simulink model "One_Sensor_Simulation"  (R2021a)
settings: Solver=FixedStepAuto  StartTime=0.0  StopTime=200  FixedStep=Ts  RelTol=1e-5
values from neighbouring files (symbols this model uses):
  accel_filter_coef = [    0.0264    0.1405    0.3331    0.3331    0.1405    0.0264]    [quad_params_ekf.m]
  g = ref_acc(3)    [ekf_measurement_jacobian.m]    (also in quad_params_ekf.m = 9.81)
  gyro_filter_den = [ 1.0000    2.2287    2.5245    1.5773    0.5410    0.0796]    [quad_params_ekf.m]
  gyro_filter_num = [ 0.2821    1.2725    2.4208    2.4208    1.2725    0.2821]    [quad_params_ekf.m]
  I = [     0.005831943165131                   0                   0 ... (first row only)    [quad_params_ekf.m]
  Kd_rates = [0.05,0.05,0.1]'    [quad_params_ekf.m]
  Kd_vel = [0.8,0.8,0.3]'    [quad_params_ekf.m]
  Ki_vel = [0.1,0.1,0.1]'    [quad_params_ekf.m]
  km = 1.2e-7    (= 1.2e-07)    [quad_params_ekf.m]
  Kp_att = [6,6,6]'    [quad_params_ekf.m]
  Kp_pos = [7,7,3]'    [quad_params_ekf.m]
  Kp_rates = [10,10,10]'    [quad_params_ekf.m]
  Kp_vel = [3,3,5]'    [quad_params_ekf.m]
  kt = 0.9e-5    (= 9e-06)    [quad_params_ekf.m]
  L = 0.2    [quad_params_ekf.m]
  m = 0.9272    [quad_params_ekf.m]
  q_init = [1;0;0;0]    [quad_params_ekf.m]
  rate_p_max = 3.5    [quad_params_ekf.m]
  thrust_max = thrust_max_per_motor*4    (= 32)    [quad_params_ekf.m]
  thrust_max_per_motor = 8    [quad_params_ekf.m]
  tilt_max = pi/6    (= 0.523598775598)    [quad_params_ekf.m]
  TQ_max_per_motor = km*(w_max.^2)    [quad_params_ekf.m]
  Ts = 0.001    [ekf_process_jacobian.m]    (also in ekf_process_model.m; quad_params_ekf.m)
  Ts_IMU = 0.001    [quad_params_ekf.m]
  Vb_init = [0;0;0]    [quad_params_ekf.m]
  vel_xy_max = 15    [quad_params_ekf.m]
  vel_z_max = 10    [quad_params_ekf.m]
  wb_init = [0;0;0]    [quad_params_ekf.m]
  Xe_init = [0;0;0]    [quad_params_ekf.m]
undefined symbols (not defined in the file or in its folder): IMU, pm_0, sigbuilder_block, Vm_0, xme_0
libraries: simulink_extras x7, aerolibutil x6, sharedutil x5, simulink x4, sharedtransform x4, pid_lib x3, aerolibcommonsys x3, aerolibnavsys x2, mspsensorlib x1, aerolibnav x1, aerolibanim x1
(part 2 of 3)

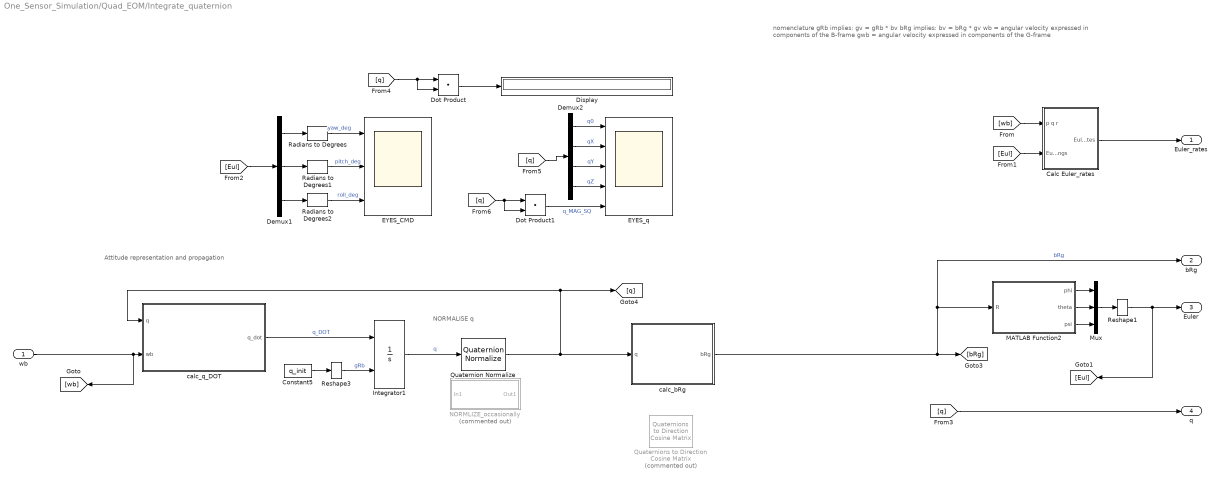
== system One_Sensor_Simulation/Quad_EOM/Integrate_quaternion ==
  note: Attitude representation and propagation
  note: nomenclature
      | gRb implies: gv = gRb * bv
      | bRg implies: bv = bRg * gv
      |
      | wb = angular velocity expressed in components of the B-frame
      | gwb = angular velocity expressed in components of the G-frame
  note: NORMALISE q
  wb : Inport
  Calc Euler_rates : Subsystem
  Constant5 : Constant  Value=q_init  OutDataTypeStr=Inherit: Inherit via back propagation
  Demux1 : Demux  Outputs=3
  Demux2 : Demux
  Display : Display
  Dot Product : DotProduct  InputSameDT=on  OutDataTypeStr=Inherit: Inherit via internal rule
  Dot Product1 : DotProduct  InputSameDT=on  OutDataTypeStr=Inherit: Inherit via internal rule
  EYES_CMD : Scope  NumInputPorts=3
  EYES_q : Scope  NumInputPorts=5
  Integrator1 : Integrator  InitialConditionSource=external
  MATLAB Function2 : MATLAB Function  TreatAsAtomicUnit=on
  Mux : Mux  Inputs=3
  NORMLIZE_occasionally : Subsystem  Commented=on
  Quaternion Normalize : sharedutil/Quaternion Normalize  aMode=aMode
      settings: SourceProductBaseCode=AE,PW,DR,MT,UV,VE
  Quaternions to Direction Cosine Matrix : sharedtransform/Quaternions to  Direction Cosine Matrix  Commented=on  aMode=aMode
      settings: SourceProductBaseCode=AE,PW,DR,MT,UV,VE
  Radians to Degrees : simulink_extras/Transformations/Radians to Degrees
  Radians to Degrees1 : simulink_extras/Transformations/Radians to Degrees
  Radians to Degrees2 : simulink_extras/Transformations/Radians to Degrees
  Reshape1 : Reshape  OutputDimensionality=Column vector (2-D)
  Reshape3 : Reshape  OutputDimensionality=Column vector (2-D)
  calc_bRg : MATLAB Function  TreatAsAtomicUnit=on
  calc_q_DOT : MATLAB Function  TreatAsAtomicUnit=on
  Euler_rates : Outport
  bRg : Outport  Port=2
  Euler : Outport  Port=3
  q : Outport  Port=4
  wires:
  Calc Euler_rates/1(Euler_rates) -> Euler_rates/1
  [Eul] -> Demux1/1
  Demux1/2 -> Radians to Degrees1/1
  Demux1/3 -> Radians to Degrees2/1
  Radians to Degrees2/1 -> EYES_CMD/3  "roll_deg"
  Radians to Degrees1/1 -> EYES_CMD/2  "pitch_deg"
  Radians to Degrees/1 -> EYES_CMD/1  "yaw_deg"
  Demux1/1 -> Radians to Degrees/1
  [Eul] -> Calc Euler_rates/2(Euler_angs)
  [wb] -> Calc Euler_rates/1("p q r ")
  Reshape1/1 -> [Eul], Euler/1
  Mux/1 -> Reshape1/1
  MATLAB Function2/3(psi) -> Mux/3
  MATLAB Function2/2(theta) -> Mux/2
  MATLAB Function2/1(phi) -> Mux/1
  Demux2/3 -> EYES_q/3  "qY"
  [q] -> Demux2/1
  Demux2/2 -> EYES_q/2  "qX"
  Demux2/1 -> EYES_q/1  "q0"
  [q] -> Dot Product1/2, Dot Product1/1
  Demux2/4 -> EYES_q/4  "qZ"
  Dot Product1/1 -> EYES_q/5  "q_MAG_SQ"
  Dot Product/1 -> Display/1
  [q] -> Dot Product/2, Dot Product/1
  Integrator1/1 -> Quaternion Normalize/1  "q"
  Quaternion Normalize/1 -> calc_bRg/1(q), [q], calc_q_DOT/1(q)
  calc_bRg/1(bRg) -> bRg/1, MATLAB Function2/1(R), [bRg]  "bRg"
  calc_q_DOT/1(q_dot) -> Integrator1/1  "q_DOT"
  Constant5/1 -> Reshape3/1
  wb/1 -> calc_q_DOT/2(wb), [wb]
  Reshape3/1 -> Integrator1/2  "gRb"
  [q] -> q/1

== system One_Sensor_Simulation/Quad_EOM/Subsystem ==
  note: I . w^' = Mb - (\omega \times (I.w))
      |
      | w^' = inv(I) * (Mb - (w \times (I.w)))
  pqr : Inport
  I : Inport  Port=2
  Moment : Inport  Port=3
  Product2 : Product  Multiplication=Matrix(*)  InputSameDT=on  SaturateOnIntegerOverflow=on  OutDataTypeStr=Inherit: Same as first input
  Product3 : Product  Inputs=/  Multiplication=Matrix(*)  SaturateOnIntegerOverflow=on  OutDataTypeStr=Inherit: Same as first input
  Product4 : Product  Multiplication=Matrix(*)  SaturateOnIntegerOverflow=on  OutDataTypeStr=Inherit: Same as first input
  Reshape10 : Reshape  OutputDimensionality=Column vector (2-D)
  Reshape8 : Reshape  OutputDimensionality=Column vector (2-D)
  Reshape9 : Reshape  OutputDimensionality=Column vector (2-D)
  Scope : Scope
  Scope1 : Scope
  Scope2 : Scope
  Sum2 : Sum  Inputs=+|-  SaturateOnIntegerOverflow=on
  w_x_(I.w) : Subsystem
      mask Display:
      | text(.5,.5,'Cross\nProduct\n\nC = AxB', ...
      | 	'HorizontalAlignment','Center',...
      | 	'VerticalAlignment','middle')
  pdot qdot rdot : Outport
  wires:
  Product2/1 -> Scope1/1, w_x_(I.w)/2(B)  "I.w"
  Product3/1 -> Product4/1  "inv(I)"
  Reshape8/1 -> Scope/1, w_x_(I.w)/1(A), Product2/2  "w"
  [I] -> Product3/1
  pqr/1 -> Reshape8/1
  Reshape9/1 -> Sum2/1  "Mb"
  Sum2/1 -> Scope2/1, Product4/2  "Mb - (w x (I.w))"
  Reshape10/1 -> Sum2/2  "w x (I.w)"
  w_x_(I.w)/1(C) -> Reshape10/1
  [I] -> Product2/1  "I"
  Product4/1 -> pdot qdot rdot/1  "w_dot"
  Moment/1 -> Reshape9/1
  I/1 -> [I]

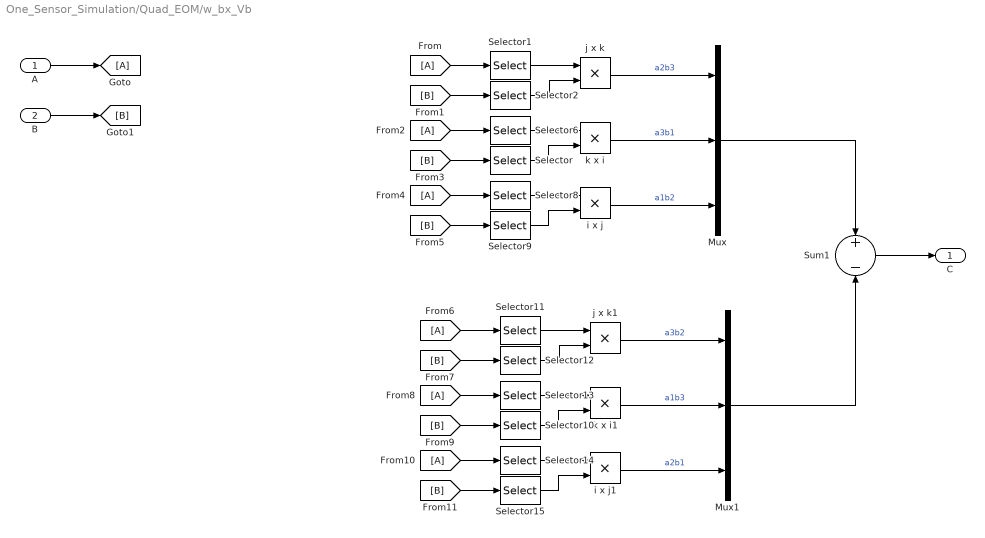
== system One_Sensor_Simulation/Quad_EOM/w_bx_Vb ==
  A : Inport
  B : Inport  Port=2
  Mux : Mux  Inputs=3
  Mux1 : Mux  Inputs=3
  Selector{,8,13,15} (4 alike) : Selector  InputPortWidth=3  IndexOptions=Index vector (dialog)  Indices=1  OutputSizes=1
  Selector{1,9,12,14} (4 alike) : Selector  InputPortWidth=3  IndexOptions=Index vector (dialog)  Indices=2  OutputSizes=1
  Selector{2,6,10..11} (4 alike) : Selector  InputPortWidth=3  IndexOptions=Index vector (dialog)  Indices=3  OutputSizes=1
  Sum1 : Sum  Inputs=+|-  InputSameDT=on  SaturateOnIntegerOverflow=on  OutDataTypeStr=Inherit: Same as first input
  i x j : Product  InputSameDT=on  SaturateOnIntegerOverflow=on  OutDataTypeStr=Inherit: Same as first input
  i x j1 : Product  InputSameDT=on  SaturateOnIntegerOverflow=on  OutDataTypeStr=Inherit: Same as first input
  j x k : Product  InputSameDT=on  SaturateOnIntegerOverflow=on  OutDataTypeStr=Inherit: Same as first input
  j x k1 : Product  InputSameDT=on  SaturateOnIntegerOverflow=on  OutDataTypeStr=Inherit: Same as first input
  k x i : Product  InputSameDT=on  SaturateOnIntegerOverflow=on  OutDataTypeStr=Inherit: Same as first input
  k x i1 : Product  InputSameDT=on  SaturateOnIntegerOverflow=on  OutDataTypeStr=Inherit: Same as first input
  C : Outport
  wires:
  i x j/1 -> Mux/3  "a1b2"
  k x i/1 -> Mux/2  "a3b1"
  j x k/1 -> Mux/1  "a2b3"
  Mux/1 -> Sum1/1
  Sum1/1 -> C/1
  Selector1/1 -> j x k/1
  Selector2/1 -> j x k/2
  B/1 -> [B]
  A/1 -> [A]
  [B] -> Selector2/1
  [A] -> Selector1/1
  [A] -> Selector6/1
  [B] -> Selector/1
  Selector6/1 -> k x i/1
  Selector/1 -> k x i/2
  [A] -> Selector8/1
  [B] -> Selector9/1
  Selector8/1 -> i x j/1
  Selector9/1 -> i x j/2
  i x j1/1 -> Mux1/3  "a2b1"
  k x i1/1 -> Mux1/2  "a1b3"
  j x k1/1 -> Mux1/1  "a3b2"
  Mux1/1 -> Sum1/2
  Selector11/1 -> j x k1/1
  Selector12/1 -> j x k1/2
  [B] -> Selector12/1
  [A] -> Selector11/1
  [A] -> Selector13/1
  [B] -> Selector10/1
  Selector13/1 -> k x i1/1
  Selector10/1 -> k x i1/2
  [A] -> Selector14/1
  [B] -> Selector15/1
  Selector14/1 -> i x j1/1
  Selector15/1 -> i x j1/2

== system One_Sensor_Simulation/Sensors and preprocessing/IMU+altitude ==
  note: Accelerometer and Gyroscope
  note: Magnetometer
  note: Altitude (not simulated)
  States : Inport
  Acc + Gyro : Subsystem  AncestorBlock=aerolibnav/Three-axis Inertial Measurement Unit  mask(Three-axis Inertial Measurement Unit){units=Metric (MKS), imu=[0 0 0], i_Ts=Ts, dtype_a=off, w_a=.7, z_a=.2, a_sf_cc=IMU.accScaleCross, a_bias=IMU.accBias, a_sat=IMU.accLimits, dtype_g=off, w_g=.7, z_g=.2, g_sf_cc=IMU.gyroScaleCross, g_bias=IMU.gyroBias, g_sens=[0, 0, 0], g_sat=IMU.gyroLimits, i_rand=on, i_seeds=IMU.noiseSeeds, i_pow=IMU.noisePower}
      mask prompts: units "aeroblks:aeroblknav:blockThreeaxisInertialMeasurementUnitParamUnits"; imu "aeroblks:aeroblknav:blockThreeaxisInertialMeasurementUnitParamIMUlocation"; i_Ts "aeroblks:aeroblknav:blockThreeaxisInertialMeasurementUnitParamUpdaterate"; dtype_a "aeroblks:aeroblknav:blockThreeaxisInertialMeasurementUnitParamSecondorderdynamicsforaccelerometer"; w_a "aeroblks:aeroblknav:blockThreeaxisInertialMeasurementUnitParamAccelerometernaturalfrequencyradsec"; z_a "aeroblks:aeroblknav:blockThreeaxisInertialMeasurementUnitParamAccelerometerdampingratio"; a_sf_cc "aeroblks:aeroblknav:blockThreeaxisInertialMeasurementUnitParamAccelerometerscalefactorandcrosscoupling"; a_bias "aeroblks:aeroblknav:blockThreeaxisInertialMeasurementUnitParamAccelerometermeasurementbias"; a_sat "aeroblks:aeroblknav:blockThreeaxisInertialMeasurementUnitParamAccelerometerupperandlowerlimits"; dtype_g "aeroblks:aeroblknav:blockThreeaxisInertialMeasurementUnitParamSecondorderdynamicsforgyro"; w_g "aeroblks:aeroblknav:blockThreeaxisInertialMeasurementUnitParamGyronaturalfrequencyradsec"; z_g "aeroblks:aeroblknav:blockThreeaxisInertialMeasurementUnitParamGyrodampingratio"; g_sf_cc "aeroblks:aeroblknav:blockThreeaxisInertialMeasurementUnitParamGyroscalefactorsandcrosscoupling"; g_bias "aeroblks:aeroblknav:blockThreeaxisInertialMeasurementUnitParamGyromeasurementbias"; g_sens "aeroblks:aeroblknav:blockThreeaxisInertialMeasurementUnitParamGsensitivebias"; g_sat "aeroblks:aeroblknav:blockThreeaxisInertialMeasurementUnitParamGyroupperandlowerlimits"; i_rand "aeroblks:aeroblknav:blockThreeaxisInertialMeasurementUnitParamNoiseon"; i_seeds "aeroblks:aeroblknav:blockThreeaxisInertialMeasurementUnitParamNoiseseeds"; i_pow "aeroblks:aeroblknav:blockThreeaxisInertialMeasurementUnitParamNoisepower"
      mask help: aeroblks:aeroblknav:blockThreeaxisInertialMeasurementUnitDesc
      mask init:
      | block = gcb;   
      | ports=aeroicon('aeroblkimu','icon');
      mask Help: eval('asbhelp');
      mask TypeOptions units: aeroblks:aeroblknav:blockThreeaxisInertialMeasurementUnitParamComboMetricMKS | aeroblks:aeroblknav:blockThreeaxisInertialMeasurementUnitParamComboEnglish
      mask Callback dtype_a: aeroicon('aeroblkimu')
      mask Callback dtype_g: aeroicon('aeroblkimu')
      mask Callback i_rand: aeroicon('aeroblkimu')
      mask DialogControl ParameterTabVar0 Prompt: Main
      mask DialogControl units Prompt: Units:
      mask DialogControl imu Prompt: IMU location:
      mask DialogControl i_Ts Prompt: Update rate:
      mask DialogControl ParameterTabVar01 Prompt: Accelerometer
      mask DialogControl dtype_a Prompt: Second-order dynamics for accelerometer
      mask DialogControl w_a Prompt: Accelerometer natural frequency (rad/sec):
      mask DialogControl z_a Prompt: Accelerometer damping ratio:
      mask DialogControl a_sf_cc Prompt: Accelerometer scale factor and cross-coupling:
      mask DialogControl a_bias Prompt: Accelerometer measurement bias:
      mask DialogControl a_sat Prompt: Accelerometer upper and lower limits:
      mask DialogControl ParameterTabVar012 Prompt: Gyroscope
      mask DialogControl dtype_g Prompt: Second-order dynamics for gyro
      mask DialogControl w_g Prompt: Gyro natural frequency (rad/sec):
      mask DialogControl z_g Prompt: Gyro damping ratio:
      mask DialogControl g_sf_cc Prompt: Gyro scale factors and cross-coupling:
      mask DialogControl g_bias Prompt: Gyro measurement bias:
      mask DialogControl g_sens Prompt: G-sensitive bias:
      mask DialogControl g_sat Prompt: Gyro upper and lower limits:
      mask DialogControl ParameterTabVar0123 Prompt: Noise
      mask DialogControl i_rand Prompt: Noise on
      mask DialogControl i_seeds Prompt: Noise seeds:
      mask DialogControl i_pow Prompt: Noise power:
      mask Display:
      | port_label(ports(1).type,ports(1).port,ports(1).txt,'texmode','on');
      | port_label(ports(2).type,ports(2).port,ports(2).txt,'texmode','on');
      | port_label(ports(3).type,ports(3).port,ports(3).txt,'texmode','on');
      | port_label(ports(4).type,ports(4).port,ports(4).txt,'texmode','on');
      | port_label(ports(5).type,ports(5).port,ports(5).txt,'texmode','on');
      | port_label(ports(6).type,ports(6).port,ports(6).txt,'texmode','on');
      | port_label(ports(7).type,ports(7).port,ports(7).txt,'texmode','on');
  Bus Selector : BusSelector  OutputSignals=Ab,wb,wb_dot
  Bus Selector1 : BusSelector  OutputSignals=Ab,bRg
  Bus Selector3 : BusSelector  OutputSignals=phi; theta; psi
  Bus Selector4 : BusSelector  OutputSignals=Xe
  Bus Selector5 : BusSelector  OutputSignals=Ab
  CG location : Constant  Value=[0, 0, 0]
  Compare yaw from mag and actual one : MATLAB Function  TreatAsAtomicUnit=on
  Gravity : Constant  Value=[0 0 -g]
  IMU : mspsensorlib/IMU  Commented=on  DispRefFrame=NED  Temperature=25  MagneticFieldNED=[ 27.5550, -2.4169, -16.0849 ]  MagneticFieldENU=[ -2.4169, 27.5550, 16.0849 ]  SeedDouble=67  SimulateUsing=Interpreted execution  AccelParamsMeasurementRange=Inf  AccelParamsResolution=0  AccelParamsConstantBias=[ 0, 0, 0 ]  AccelParamsAxesMisalignment=[ 0, 0, 0 ]  AccelParamsNoiseDensity=[ 0, 0, 0 ]  AccelParamsBiasInstability=[ 0, 0, 0 ]  AccelParamsRandomWalk=[ 0, 0, 0 ]  AccelParamsTemperatureBias=[ 0, 0, 0 ]  AccelParamsTemperatureScaleFactor=[ 0, 0, 0 ]  GyroParamsMeasurementRange=Inf  GyroParamsResolution=0  GyroParamsConstantBias=[ 0, 0, 0 ]  GyroParamsAxesMisalignment=[ 0, 0, 0 ]  GyroParamsAccelerationBias=[ 0, 0, 0 ]  GyroParamsNoiseDensity=[ 0, 0, 0 ]  GyroParamsBiasInstability=[ 0, 0, 0 ]  GyroParamsRandomWalk=[ 0, 0, 0 ]  GyroParamsTemperatureBias=[ 0, 0, 0 ]  GyroParamsTemperatureScaleFactor=[ 0, 0, 0 ]  MagParamsMeasurementRange=Inf  MagParamsResolution=0  MagParamsConstantBias=[ 0, 0, 0 ]  MagParamsAxesMisalignment=[ 0, 0, 0 ]  MagParamsNoiseDensity=[ 0, 0, 0 ]  MagParamsBiasInstability=[ 0, 0, 0 ]  MagParamsRandomWalk=[ 0, 0, 0 ]  MagParamsTemperatureBias=[ 0, 0, 0 ]  MagParamsTemperatureScaleFactor=[ 0, 0, 0 ]
      settings: SourceProductBaseCode=TF,NV
  Magnetometer : Subsystem
  Mux : Mux  Inputs=2
  Scope : Scope
  Selector : Selector  InputPortWidth=3  IndexOptions=Index vector (dialog)  Indices=[3]  OutputSizes=1
  Selector2 : Selector  InputPortWidth=3  IndexOptions=Index vector (dialog)  Indices=[3]  OutputSizes=1
  Three-axis Inertial Measurement Unit1 : aerolibnav/Three-axis Inertial Measurement Unit  Commented=on  units=Metric (MKS)  imu=[0 0 0]  i_Ts=Ts_IMU  dtype_a=on  w_a=190  z_a=0.707  a_sf_cc=[1 0 0; 0 1 0; 0 0 1]  a_bias=[0 0 0]  a_sat="[-inf  -inf  -inf  inf inf inf]"  dtype_g=on  w_g=190  z_g=0.707  g_sf_cc=[1 0 0; 0 1 0; 0 0 1]  g_bias=[0 0 0]  g_sens=[0 0 0]  g_sat="[-inf  -inf  -inf  inf inf inf]"  i_rand=on  i_seeds=[23093 23094 23095 23096 23097 23098]  i_pow=[0.001 0.001 0.001 0.0001 0.0001 0.0001]
  acc : Outport
  gyro : Outport  Port=2
  alt : Outport  Port=3
  mag : Outport  Port=4
  wires:
  Selector2/1 -> alt/1  "altitude"
  CG location/1 -> Acc + Gyro/4(CG)
  Bus Selector/3 -> Acc + Gyro/3(w_dot)  "<wb_dot>"
  Bus Selector/2 -> Acc + Gyro/2(w)  "<wb>"
  Bus Selector/1 -> Acc + Gyro/1(A_b)  "<Ab>"
  Acc + Gyro/2(w_meas) -> gyro/1  "gyro"
  Gravity/1 -> Acc + Gyro/5(g)  "Gravity_ned"
  Acc + Gyro/1(A_meas) -> acc/1  "acc"
  Selector/1 -> Mux/2  "yaw"
  Compare yaw from mag and actual one/1(yaw) -> Mux/1
  Mux/1 -> Scope/1
  Bus Selector1/2 -> Magnetometer/2(<bRg>)  "<bRg>"
  Magnetometer/1(mag) -> mag/1, Compare yaw from mag and actual one/2(mag_vec)
  States/1 -> [states]
  [states] -> Bus Selector/1
  [states] -> Bus Selector1/1
  [states] -> Bus Selector3/1
  Bus Selector3/1 -> Selector/1  "<phi; theta; psi>"
  [states] -> Bus Selector4/1
  Bus Selector4/1 -> Selector2/1  "<Xe>"
  Bus Selector1/1 -> Magnetometer/1(acc)  "<Ab>"
  [states] -> Bus Selector5/1
  Bus Selector5/1 -> Compare yaw from mag and actual one/1(acc_vec)  "<Ab>"

== system One_Sensor_Simulation/Sensors and preprocessing/Preprocessing and Filtering ==
  acc_raw : Inport
  gyro_raw : Inport  Port=2
  alt_raw : Inport  Port=3
  mag_raw : Inport  Port=4
  Cast To Double{,1..2,4} (4 alike) : DataTypeConversion  OutDataTypeStr=double
  Constant : Constant  Value=[0 0 g]
  FIR_IMUaccel : DiscreteFir  Coefficients=accel_filter_coef
  IIR_IMUgyro : DiscreteFilter  Numerator=gyro_filter_num  Denominator=gyro_filter_den
  Sum : Sum  Inputs=-+|
  Sum1 : Sum  Inputs=-+|
  Sum2 : Sum  Inputs=-+|
  Sum3 : Sum  Inputs=|+-
  bias : Constant  Value=IMU.accBiasEst
  filtering : Subsystem
  gyro bias : Constant  Value=IMU.gyroBiasEst
  inverseI_acc_gain : Gain  Gain=IMU.inverseAccGain  ParamDataTypeStr=single  OutDataTypeStr=single
  inverseI_gyro_gain : Gain  Gain=IMU.inverseGyroGain  ParamDataTypeStr=single  OutDataTypeStr=single
  inverseI_mag_gain : Gain  Gain=IMU.inverseMagGain  ParamDataTypeStr=single  OutDataTypeStr=single
  mag bias : Constant  Value=IMU.magBiasEst
  acc_zero : Outport
  acc : Outport  Port=2
  gyro : Outport  Port=3
  alt : Outport  Port=4
  mag : Outport  Port=5
  wires:
  gyro bias/1 -> Sum2/1
  Cast To Double/1 -> acc/1, Sum/2  "acc"
  bias/1 -> Sum1/1
  mag bias/1 -> Sum3/2
  FIR_IMUaccel/1 -> Cast To Double/1  "acc"
  inverseI_gyro_gain/1 -> filtering/1(gyro_raw)  "gyro"
  mag_raw/1 -> Sum3/1
  Sum3/1 -> inverseI_mag_gain/1  "gyro"
  Sum1/1 -> inverseI_acc_gain/1  "acc"
  Sum/1 -> acc_zero/1  "acc_zero"
  Sum2/1 -> inverseI_gyro_gain/1  "gyro"
  Cast To Double1/1 -> gyro/1  "gyro"
  inverseI_mag_gain/1 -> IIR_IMUgyro/1  "mag"
  IIR_IMUgyro/1 -> Cast To Double4/1
  filtering/1(gyro) -> Cast To Double1/1  "gyro"
  inverseI_acc_gain/1 -> FIR_IMUaccel/1  "acc"
  Cast To Double4/1 -> mag/1  "mag"
  Constant/1 -> Sum/1
  acc_raw/1 -> Sum1/2
  gyro_raw/1 -> Sum2/2
  Cast To Double2/1 -> alt/1  "alt"
  alt_raw/1 -> Cast To Double2/1

== system One_Sensor_Simulation/Trajectory command/Altitude ==
  "Altitude " : Subsystem  Tag=STV Subsys  LoadFcn=sigbuilder_block('load');  StartFcn=sigbuilder_block('start');  StopFcn=sigbuilder_block('stop');  ClipboardFcn=sigbuilder_block('clipboard');  VariantControl=Choice_1  mask(Sigbuilder block){tuvar=[0:10]}
      mask help: Simulink:masks:SigbuilderBlock_MD
      mask init:
      | if ~strcmp(get_param(bdroot(gcbh),'SimulationStatus'),'stopped') tuvar = sigbuilder_block('maskInit'); end
      settings: CopyFcn=sigbuilder_block('copy');  DeleteFcn=sigbuilder_block('delete');  ModelCloseFcn=sigbuilder_block('modelClose');  PreSaveFcn=sigbuilder_block('preSave');  PauseFcn=sigbuilder_block('pause');  ContinueFcn=sigbuilder_block('continue');  NameChangeFcn=sigbuilder_block('namechange');  OpenFcn=sigbuilder_block('open',[200.1 155.1 551.4 400.5 ]);  CloseFcn=sigbuilder_block('close');
      mask Display: plot(0, 0, 100, 100,[2, 2, 32, 32, 2], [68, 8, 8, 68, 68],[32, 2], [38, 38], [32, 19, 2],[53, 60, 44], [32, 17, 17, 2],[16, 16, 31, 31]);txt = getActiveGroup(gcbh);text(2, 100, txt,'verticalAlignment', 'top');
  Bus Creator : BusCreator  Inputs=4
  Z : Outport
  Y : Outport  Port=2
  X : Outport  Port=3
  Yaw : Outport  Port=4
  CMD_VEC : Outport  Port=5
  wires:
  "Altitude "/4(Yaw) -> Bus Creator/1, Yaw/1  "yaw_cmd"
  "Altitude "/2(Y) -> Bus Creator/3, Y/1  "y_cmd"
  "Altitude "/1(Z) -> Bus Creator/4, Z/1  "z_cmd"
  "Altitude "/3(X) -> Bus Creator/2, X/1  "x_cmd"
  Bus Creator/1 -> CMD_VEC/1

== system One_Sensor_Simulation/Trajectory command/Ground ==
  Bus Creator : BusCreator  Inputs=4
  Zero{,1..3} (4 alike) : Constant  Value=0  OutDataTypeStr=Inherit: Inherit via back propagation
  Z : Outport
  Y : Outport  Port=2
  X : Outport  Port=3
  Yaw : Outport  Port=4
  CMD_VEC : Outport  Port=5
  wires:
  Zero3/1 -> Bus Creator/1, Yaw/1  "yaw_cmd"
  Zero2/1 -> Bus Creator/3, Y/1  "y_cmd"
  Zero/1 -> Bus Creator/4, Z/1  "z_cmd"
  Zero1/1 -> Bus Creator/2, X/1  "x_cmd"
  Bus Creator/1 -> CMD_VEC/1

== system One_Sensor_Simulation/Trajectory command/Position Trajectory ==
  Bus Creator : BusCreator  Inputs=4
  Degrees to Radians : simulink_extras/Transformations/Degrees to Radians
  multisteps : Subsystem  Tag=STV Subsys  LoadFcn=sigbuilder_block('load');  StartFcn=sigbuilder_block('start');  StopFcn=sigbuilder_block('stop');  ClipboardFcn=sigbuilder_block('clipboard');  VariantControl=Choice_5  mask(Sigbuilder block){tuvar=[0:10]}
      mask help: Simulink:masks:SigbuilderBlock_MD
      mask init:
      | if ~strcmp(get_param(bdroot(gcbh),'SimulationStatus'),'stopped') tuvar = sigbuilder_block('maskInit'); end
      settings: CopyFcn=sigbuilder_block('copy');  DeleteFcn=sigbuilder_block('delete');  ModelCloseFcn=sigbuilder_block('modelClose');  PreSaveFcn=sigbuilder_block('preSave');  PauseFcn=sigbuilder_block('pause');  ContinueFcn=sigbuilder_block('continue');  NameChangeFcn=sigbuilder_block('namechange');  OpenFcn=sigbuilder_block('open',[4.8 36 1142.4 525.6 ]);  CloseFcn=sigbuilder_block('close');
      mask Display: plot(0, 0, 100, 100,[2, 2, 32, 32, 2], [68, 8, 8, 68, 68],[32, 2], [38, 38], [32, 19, 2],[53, 60, 44], [32, 17, 17, 2],[16, 16, 31, 31]);txt = getActiveGroup(gcbh);text(2, 100, txt,'verticalAlignment', 'top');
  Z : Outport
  Y : Outport  Port=2
  X : Outport  Port=3
  Yaw : Outport  Port=4
  CMD_VEC : Outport  Port=5
  wires:
  Degrees to Radians/1 -> Bus Creator/1, Yaw/1  "yaw_cmd"
  multisteps/2(Y) -> Bus Creator/3, Y/1  "y_cmd"
  multisteps/1(Z) -> Bus Creator/4, Z/1  "z_cmd"
  multisteps/3(X) -> Bus Creator/2, X/1  "x_cmd"
  Bus Creator/1 -> CMD_VEC/1
  multisteps/4(Yaw) -> Degrees to Radians/1  "yaw_cmd"

== system One_Sensor_Simulation/Trajectory command/Test to visualize thrust dir ==
  Bus Creator : BusCreator  Inputs=4
  multisteps : Subsystem  Tag=STV Subsys  LoadFcn=sigbuilder_block('load');  StartFcn=sigbuilder_block('start');  StopFcn=sigbuilder_block('stop');  ClipboardFcn=sigbuilder_block('clipboard');  VariantControl=Choice_5  mask(Sigbuilder block){tuvar=[0:10]}
      mask help: Simulink:masks:SigbuilderBlock_MD
      mask init:
      | if ~strcmp(get_param(bdroot(gcbh),'SimulationStatus'),'stopped') tuvar = sigbuilder_block('maskInit'); end
      settings: CopyFcn=sigbuilder_block('copy');  DeleteFcn=sigbuilder_block('delete');  ModelCloseFcn=sigbuilder_block('modelClose');  PreSaveFcn=sigbuilder_block('preSave');  PauseFcn=sigbuilder_block('pause');  ContinueFcn=sigbuilder_block('continue');  NameChangeFcn=sigbuilder_block('namechange');  OpenFcn=sigbuilder_block('open',[0 36 1152 560.4 ]);  CloseFcn=sigbuilder_block('close');
      mask Display: plot(0, 0, 100, 100,[2, 2, 32, 32, 2], [68, 8, 8, 68, 68],[32, 2], [38, 38], [32, 19, 2],[53, 60, 44], [32, 17, 17, 2],[16, 16, 31, 31]);txt = getActiveGroup(gcbh);text(2, 100, txt,'verticalAlignment', 'top');
  Z : Outport
  Y : Outport  Port=2
  X : Outport  Port=3
  Yaw : Outport  Port=4
  CMD_VEC : Outport  Port=5
  wires:
  multisteps/2(Y) -> Bus Creator/3, Y/1  "y_cmd"
  multisteps/1(Z) -> Bus Creator/4, Z/1  "z_cmd"
  multisteps/3(X) -> Bus Creator/2, X/1  "x_cmd"
  Bus Creator/1 -> CMD_VEC/1
  multisteps/4(Yaw) -> Bus Creator/1, Yaw/1  "yaw_cmd"

== system One_Sensor_Simulation/Trajectory command/X Sine ==
  Bus Creator : BusCreator  Inputs=4
  sine wave on X : Subsystem  Tag=STV Subsys  LoadFcn=sigbuilder_block('load');  StartFcn=sigbuilder_block('start');  StopFcn=sigbuilder_block('stop');  ClipboardFcn=sigbuilder_block('clipboard');  VariantControl=Choice_3  mask(Sigbuilder block){tuvar=[0:10]}
      mask help: Simulink:masks:SigbuilderBlock_MD
      mask init:
      | if ~strcmp(get_param(bdroot(gcbh),'SimulationStatus'),'stopped') tuvar = sigbuilder_block('maskInit'); end
      settings: CopyFcn=sigbuilder_block('copy');  DeleteFcn=sigbuilder_block('delete');  ModelCloseFcn=sigbuilder_block('modelClose');  PreSaveFcn=sigbuilder_block('preSave');  PauseFcn=sigbuilder_block('pause');  ContinueFcn=sigbuilder_block('continue');  NameChangeFcn=sigbuilder_block('namechange');  OpenFcn=sigbuilder_block('open',[452.4 149.7 551.4 400.5 ]);  CloseFcn=sigbuilder_block('close');
      mask Display: plot(0, 0, 100, 100,[2, 2, 32, 32, 2], [68, 8, 8, 68, 68],[32, 2], [38, 38], [32, 19, 2],[53, 60, 44], [32, 17, 17, 2],[16, 16, 31, 31]);txt = getActiveGroup(gcbh);text(2, 100, txt,'verticalAlignment', 'top');
  Z : Outport
  Y : Outport  Port=2
  X : Outport  Port=3
  Yaw : Outport  Port=4
  CMD_VEC : Outport  Port=5
  wires:
  sine wave on X/4(Yaw) -> Bus Creator/1, Yaw/1  "yaw_cmd"
  sine wave on X/2(Y) -> Bus Creator/3, Y/1  "y_cmd"
  sine wave on X/1(Z) -> Bus Creator/4, Z/1  "z_cmd"
  sine wave on X/3(X) -> Bus Creator/2, X/1  "x_cmd"
  Bus Creator/1 -> CMD_VEC/1

== system One_Sensor_Simulation/Trajectory command/X ramp ==
  " ramp on X" : Subsystem  Tag=STV Subsys  LoadFcn=sigbuilder_block('load');  StartFcn=sigbuilder_block('start');  StopFcn=sigbuilder_block('stop');  ClipboardFcn=sigbuilder_block('clipboard');  VariantControl=Choice_3  mask(Sigbuilder block){tuvar=[0:10]}
      mask help: Simulink:masks:SigbuilderBlock_MD
      mask init:
      | if ~strcmp(get_param(bdroot(gcbh),'SimulationStatus'),'stopped') tuvar = sigbuilder_block('maskInit'); end
      settings: CopyFcn=sigbuilder_block('copy');  DeleteFcn=sigbuilder_block('delete');  ModelCloseFcn=sigbuilder_block('modelClose');  PreSaveFcn=sigbuilder_block('preSave');  PauseFcn=sigbuilder_block('pause');  ContinueFcn=sigbuilder_block('continue');  NameChangeFcn=sigbuilder_block('namechange');  OpenFcn=sigbuilder_block('open',[76.2 101.7 551.4 400.5 ]);  CloseFcn=sigbuilder_block('close');
      mask Display: plot(0, 0, 100, 100,[2, 2, 32, 32, 2], [68, 8, 8, 68, 68],[32, 2], [38, 38], [32, 19, 2],[53, 60, 44], [32, 17, 17, 2],[16, 16, 31, 31]);txt = getActiveGroup(gcbh);text(2, 100, txt,'verticalAlignment', 'top');
  Bus Creator : BusCreator  Inputs=4
  Z : Outport
  Y : Outport  Port=2
  X : Outport  Port=3
  Yaw : Outport  Port=4
  CMD_VEC : Outport  Port=5
  wires:
  " ramp on X"/4(Yaw) -> Bus Creator/1, Yaw/1  "yaw_cmd"
  " ramp on X"/2(Y) -> Bus Creator/3, Y/1  "y_cmd"
  " ramp on X"/1(Z) -> Bus Creator/4, Z/1  "z_cmd"
  " ramp on X"/3(X) -> Bus Creator/2, X/1  "x_cmd"
  Bus Creator/1 -> CMD_VEC/1

== system One_Sensor_Simulation/Trajectory command/X square ==
  Bus Creator : BusCreator  Inputs=4
  sine wave on X : Subsystem  Tag=STV Subsys  LoadFcn=sigbuilder_block('load');  StartFcn=sigbuilder_block('start');  StopFcn=sigbuilder_block('stop');  ClipboardFcn=sigbuilder_block('clipboard');  VariantControl=Choice_3  mask(Sigbuilder block){tuvar=[0:10]}
      mask help: Simulink:masks:SigbuilderBlock_MD
      mask init:
      | if ~strcmp(get_param(bdroot(gcbh),'SimulationStatus'),'stopped') tuvar = sigbuilder_block('maskInit'); end
      settings: CopyFcn=sigbuilder_block('copy');  DeleteFcn=sigbuilder_block('delete');  ModelCloseFcn=sigbuilder_block('modelClose');  PreSaveFcn=sigbuilder_block('preSave');  PauseFcn=sigbuilder_block('pause');  ContinueFcn=sigbuilder_block('continue');  NameChangeFcn=sigbuilder_block('namechange');  OpenFcn=sigbuilder_block('open',[452.4 149.7 551.4 400.5 ]);  CloseFcn=sigbuilder_block('close');
      mask Display: plot(0, 0, 100, 100,[2, 2, 32, 32, 2], [68, 8, 8, 68, 68],[32, 2], [38, 38], [32, 19, 2],[53, 60, 44], [32, 17, 17, 2],[16, 16, 31, 31]);txt = getActiveGroup(gcbh);text(2, 100, txt,'verticalAlignment', 'top');
  Z : Outport
  Y : Outport  Port=2
  X : Outport  Port=3
  Yaw : Outport  Port=4
  CMD_VEC : Outport  Port=5
  wires:
  sine wave on X/4(Yaw) -> Bus Creator/1, Yaw/1  "yaw_cmd"
  sine wave on X/2(Y) -> Bus Creator/3, Y/1  "y_cmd"
  sine wave on X/1(Z) -> Bus Creator/4, Z/1  "z_cmd"
  sine wave on X/3(X) -> Bus Creator/2, X/1  "x_cmd"
  Bus Creator/1 -> CMD_VEC/1

== system One_Sensor_Simulation/Trajectory command/Y Sine ==
  Bus Creator : BusCreator  Inputs=4
  sine wave on Y : Subsystem  Tag=STV Subsys  LoadFcn=sigbuilder_block('load');  StartFcn=sigbuilder_block('start');  StopFcn=sigbuilder_block('stop');  ClipboardFcn=sigbuilder_block('clipboard');  VariantControl=Choice_3  mask(Sigbuilder block){tuvar=[0:10]}
      mask help: Simulink:masks:SigbuilderBlock_MD
      mask init:
      | if ~strcmp(get_param(bdroot(gcbh),'SimulationStatus'),'stopped') tuvar = sigbuilder_block('maskInit'); end
      settings: CopyFcn=sigbuilder_block('copy');  DeleteFcn=sigbuilder_block('delete');  ModelCloseFcn=sigbuilder_block('modelClose');  PreSaveFcn=sigbuilder_block('preSave');  PauseFcn=sigbuilder_block('pause');  ContinueFcn=sigbuilder_block('continue');  NameChangeFcn=sigbuilder_block('namechange');  OpenFcn=sigbuilder_block('open',[4.8 36 1142.4 525.6 ]);  CloseFcn=sigbuilder_block('close');
      mask Display: plot(0, 0, 100, 100,[2, 2, 32, 32, 2], [68, 8, 8, 68, 68],[32, 2], [38, 38], [32, 19, 2],[53, 60, 44], [32, 17, 17, 2],[16, 16, 31, 31]);txt = getActiveGroup(gcbh);text(2, 100, txt,'verticalAlignment', 'top');
  Z : Outport
  Y : Outport  Port=2
  X : Outport  Port=3
  Yaw : Outport  Port=4
  CMD_VEC : Outport  Port=5
  wires:
  sine wave on Y/4(Yaw) -> Bus Creator/1, Yaw/1  "yaw_cmd"
  sine wave on Y/2(Y) -> Bus Creator/3, Y/1  "y_cmd"
  sine wave on Y/1(Z) -> Bus Creator/4, Z/1  "z_cmd"
  sine wave on Y/3(X) -> Bus Creator/2, X/1  "x_cmd"
  Bus Creator/1 -> CMD_VEC/1

== system One_Sensor_Simulation/Trajectory command/Y ramp ==
  Bus Creator : BusCreator  Inputs=4
  square on Y : Subsystem  Tag=STV Subsys  LoadFcn=sigbuilder_block('load');  StartFcn=sigbuilder_block('start');  StopFcn=sigbuilder_block('stop');  ClipboardFcn=sigbuilder_block('clipboard');  VariantControl=Choice_3  mask(Sigbuilder block){tuvar=[0:10]}
      mask help: Simulink:masks:SigbuilderBlock_MD
      mask init:
      | if ~strcmp(get_param(bdroot(gcbh),'SimulationStatus'),'stopped') tuvar = sigbuilder_block('maskInit'); end
      settings: CopyFcn=sigbuilder_block('copy');  DeleteFcn=sigbuilder_block('delete');  ModelCloseFcn=sigbuilder_block('modelClose');  PreSaveFcn=sigbuilder_block('preSave');  PauseFcn=sigbuilder_block('pause');  ContinueFcn=sigbuilder_block('continue');  NameChangeFcn=sigbuilder_block('namechange');  OpenFcn=sigbuilder_block('open',[4.8 36 1142.4 525.6 ]);  CloseFcn=sigbuilder_block('close');
      mask Display: plot(0, 0, 100, 100,[2, 2, 32, 32, 2], [68, 8, 8, 68, 68],[32, 2], [38, 38], [32, 19, 2],[53, 60, 44], [32, 17, 17, 2],[16, 16, 31, 31]);txt = getActiveGroup(gcbh);text(2, 100, txt,'verticalAlignment', 'top');
  Z : Outport
  Y : Outport  Port=2
  X : Outport  Port=3
  Yaw : Outport  Port=4
  CMD_VEC : Outport  Port=5
  wires:
  square on Y/4(Yaw) -> Bus Creator/1, Yaw/1  "yaw_cmd"
  square on Y/2(Y) -> Bus Creator/3, Y/1  "y_cmd"
  square on Y/1(Z) -> Bus Creator/4, Z/1  "z_cmd"
  square on Y/3(X) -> Bus Creator/2, X/1  "x_cmd"
  Bus Creator/1 -> CMD_VEC/1

== system One_Sensor_Simulation/Trajectory command/Yaw Sine ==
  Bus Creator : BusCreator  Inputs=4
  yaw : Subsystem  Tag=STV Subsys  LoadFcn=sigbuilder_block('load');  StartFcn=sigbuilder_block('start');  StopFcn=sigbuilder_block('stop');  ClipboardFcn=sigbuilder_block('clipboard');  VariantControl=Choice_4  mask(Sigbuilder block){tuvar=[0:10]}
      mask help: Simulink:masks:SigbuilderBlock_MD
      mask init:
      | if ~strcmp(get_param(bdroot(gcbh),'SimulationStatus'),'stopped') tuvar = sigbuilder_block('maskInit'); end
      settings: CopyFcn=sigbuilder_block('copy');  DeleteFcn=sigbuilder_block('delete');  ModelCloseFcn=sigbuilder_block('modelClose');  PreSaveFcn=sigbuilder_block('preSave');  PauseFcn=sigbuilder_block('pause');  ContinueFcn=sigbuilder_block('continue');  NameChangeFcn=sigbuilder_block('namechange');  OpenFcn=sigbuilder_block('open',[452.4 149.7 551.4 400.5 ]);  CloseFcn=sigbuilder_block('close');
      mask Display: plot(0, 0, 100, 100,[2, 2, 32, 32, 2], [68, 8, 8, 68, 68],[32, 2], [38, 38], [32, 19, 2],[53, 60, 44], [32, 17, 17, 2],[16, 16, 31, 31]);txt = getActiveGroup(gcbh);text(2, 100, txt,'verticalAlignment', 'top');
  Z : Outport
  Y : Outport  Port=2
  X : Outport  Port=3
  Yaw : Outport  Port=4
  CMD_VEC : Outport  Port=5
  wires:
  yaw/4(Yaw) -> Bus Creator/1, Yaw/1  "yaw_cmd"
  yaw/2(Y) -> Bus Creator/3, Y/1  "y_cmd"
  yaw/1(Z) -> Bus Creator/4, Z/1  "z_cmd"
  yaw/3(X) -> Bus Creator/2, X/1  "x_cmd"
  Bus Creator/1 -> CMD_VEC/1

== system One_Sensor_Simulation/Trajectory command/Yaw steps ==
  Bus Creator : BusCreator  Inputs=4
  yaw steps : Subsystem  Tag=STV Subsys  LoadFcn=sigbuilder_block('load');  StartFcn=sigbuilder_block('start');  StopFcn=sigbuilder_block('stop');  ClipboardFcn=sigbuilder_block('clipboard');  VariantControl=Choice_4  mask(Sigbuilder block){tuvar=[0:10]}
      mask help: Simulink:masks:SigbuilderBlock_MD
      mask init:
      | if ~strcmp(get_param(bdroot(gcbh),'SimulationStatus'),'stopped') tuvar = sigbuilder_block('maskInit'); end
      settings: CopyFcn=sigbuilder_block('copy');  DeleteFcn=sigbuilder_block('delete');  ModelCloseFcn=sigbuilder_block('modelClose');  PreSaveFcn=sigbuilder_block('preSave');  PauseFcn=sigbuilder_block('pause');  ContinueFcn=sigbuilder_block('continue');  NameChangeFcn=sigbuilder_block('namechange');  OpenFcn=sigbuilder_block('open',[452.4 149.7 551.4 400.5 ]);  CloseFcn=sigbuilder_block('close');
      mask Display: plot(0, 0, 100, 100,[2, 2, 32, 32, 2], [68, 8, 8, 68, 68],[32, 2], [38, 38], [32, 19, 2],[53, 60, 44], [32, 17, 17, 2],[16, 16, 31, 31]);txt = getActiveGroup(gcbh);text(2, 100, txt,'verticalAlignment', 'top');
  Z : Outport
  Y : Outport  Port=2
  X : Outport  Port=3
  Yaw : Outport  Port=4
  CMD_VEC : Outport  Port=5
  wires:
  yaw steps/4(Yaw) -> Bus Creator/1, Yaw/1  "yaw_cmd"
  yaw steps/2(Y) -> Bus Creator/3, Y/1  "y_cmd"
  yaw steps/1(Z) -> Bus Creator/4, Z/1  "z_cmd"
  yaw steps/3(X) -> Bus Creator/2, X/1  "x_cmd"
  Bus Creator/1 -> CMD_VEC/1

== system One_Sensor_Simulation/Control allocation and motor control/Ideal Actuators with allocation/Control allocation ==
  note: $C^{-1} = \left(\begin{array}{cccc} \frac{1}{4\,\mathrm{kt}} & 0 & \frac{1}{2\,L\,\mathrm{kt}} & -\frac{1}{4\,\mathrm{km}}\\ \frac{1}{4\,\mathrm{kt}} & -\frac{1}{2\,L\,\mathrm{kt}} & 0 & \frac{1}{4\,\mathrm{km}}\\ \frac{1}{4\,\mathrm{kt}} & 0 & -\frac{1}{2\,L\,\mathrm{kt}} & -\frac{1}{4\,\mathrm{km}}\\ \frac{1}{4\,\mathrm{kt}} & \frac{1}{2\,L\,\mathrm{kt}} & 0 & \frac{1}{4\,\mathrm{km}} \end{array}\right)$
  note: THRUST = k_t . \omega^2
      |
      | TORQUE = k_m . \omega^2
  THRUST_CMD : Inport
  TQ_Roll_CMD : Inport  Port=2
  TQ_Pitch_CMD : Inport  Port=3
  TQ_Yaw_CMD : Inport  Port=4
  CMD F_and_M and wRPS : Scope  NumInputPorts=8
  Constant : Constant  Value=kt
  Constant1 : Constant  Value=km
  Constant2 : Constant  Value=L
  Demux1 : Demux
  Demux2 : Demux
  Demux3 : Demux
  FM_to_w2 : MATLAB Function  TreatAsAtomicUnit=on
  Mux : Mux
  Scope : Scope
  Sqrt : Sqrt  SaturateOnIntegerOverflow=on
  Subsystem : Subsystem
  W2_checker : Subsystem
  w_command : Outport  VectorParamsAs1DForOutWhenUnconnected=off
  wires:
  Constant1/1 -> FM_to_w2/3(km)
  Constant/1 -> FM_to_w2/2(kt)
  Constant2/1 -> FM_to_w2/1(L)
  FM_to_w2/1(w2_cmd) -> Scope/1, W2_checker/1(w2_CMD)
  Sqrt/1 -> w_command/1, [w_CMD]  "w"
  W2_checker/1(w2) -> Sqrt/1
  Demux1/1 -> FM_to_w2/4(Thrust)
  Demux1/2 -> FM_to_w2/5(M_x)
  Demux1/3 -> FM_to_w2/6(M_y)
  Demux1/4 -> FM_to_w2/7(M_z)
  THRUST_CMD/1 -> Mux/1
  TQ_Roll_CMD/1 -> Mux/2
  TQ_Pitch_CMD/1 -> Mux/3
  TQ_Yaw_CMD/1 -> Mux/4
  Mux/1 -> [FM_CMD]
  [FM_CMD] -> Demux1/1
  Demux2/1 -> CMD F_and_M and wRPS/1  "Thrust"
  Demux2/2 -> CMD F_and_M and wRPS/2  "TQ_Roll_X"
  Demux2/3 -> CMD F_and_M and wRPS/3  "TQ_Pitch_Y"
  Demux2/4 -> CMD F_and_M and wRPS/4  "TQ_Yaw_Z"
  Demux3/2 -> CMD F_and_M and wRPS/6  "w2_RPS"
  Demux3/1 -> CMD F_and_M and wRPS/5  "w1_RPS"
  Demux3/4 -> CMD F_and_M and wRPS/8  "w4_RPS"
  Demux3/3 -> CMD F_and_M and wRPS/7  "w3_RPS"
  [FM_CMD] -> Demux2/1
  Subsystem/1(RPS) -> Demux3/1
  [w_CMD] -> Subsystem/1(w_per_sec)

== system One_Sensor_Simulation/Control allocation and motor control/Ideal Actuators with allocation/Perfect actuators ==
  w_cmd : Inport
  Allocation matrix (motor speed to twist) : MATLAB Function  TreatAsAtomicUnit=on
  Constant3 : Constant  Value=kt
  Constant4 : Constant  Value=km
  Constant5 : Constant  Value=L
  Demux : Demux
  Math Function1 : Math  Operator=square  SignedPower=on  SaturateOnIntegerOverflow=on
  Motor Control : Subsystem
      mask Display: image('$imagefile'); % Use "Edit Image" on toolstrip to change.
  Mux1 : Mux
  Reshape1 : Reshape  OutputDimensionality=Column vector (2-D)
  Thrust : Outport  VectorParamsAs1DForOutWhenUnconnected=off
  Mx : Outport  Port=2  VectorParamsAs1DForOutWhenUnconnected=off
  My : Outport  Port=3  VectorParamsAs1DForOutWhenUnconnected=off
  Mz : Outport  Port=4  VectorParamsAs1DForOutWhenUnconnected=off
  T_actual : Outport  Port=5  VectorParamsAs1DForOutWhenUnconnected=off
  w_mot_actual : Outport  Port=6  VectorParamsAs1DForOutWhenUnconnected=off
  wires:
  Demux/2 -> Mx/1
  Demux/1 -> Thrust/1
  Demux/3 -> My/1
  Demux/4 -> Mz/1
  [FM] -> Demux/1
  Constant3/1 -> Allocation matrix (motor speed to twist)/2(kt)
  Mux1/1 -> [FM]
  Allocation matrix (motor speed to twist)/4(M_z) -> Mux1/4
  Allocation matrix (motor speed to twist)/1(Thrust) -> Mux1/1
  Allocation matrix (motor speed to twist)/2(M_x) -> Mux1/2
  Allocation matrix (motor speed to twist)/3(M_y) -> Mux1/3
  Constant4/1 -> Allocation matrix (motor speed to twist)/3(km)
  [FM] -> T_actual/1
  Constant5/1 -> Allocation matrix (motor speed to twist)/1(L)
  Math Function1/1 -> Allocation matrix (motor speed to twist)/4(w2_col)
  Reshape1/1 -> Math Function1/1
  Motor Control/1(w) -> w_mot_actual/1, Reshape1/1  "w_actual"
  w_cmd/1 -> Motor Control/1(w_CMD)

== system One_Sensor_Simulation/Quad with sensors/Integrate_quaternion/Calc Euler_rates ==
  "p q r " : Inport
  Euler_angs : Inport  Port=2
  Demux1 : Demux  Outputs=3
  Demux2 : Demux  Outputs=3
  Demux3 : Demux  Outputs=3
  Mux1 : Mux  Inputs=3
  Reshape1 : Reshape  OutputDimensionality=Column vector (2-D)
  Reshape2 : Reshape  OutputDimensionality=Column vector (2-D)
  Terminator : Terminator
  euler_rates : MATLAB Function  TreatAsAtomicUnit=on
  Euler_rates : Outport
  wires:
  Demux2/2 -> Mux1/2  "thetadot_Y2_pitch"
  Demux1/1 -> euler_rates/1(phi_t)  "phi"
  Demux3/2 -> euler_rates/4(q)
  Demux2/1 -> Mux1/1  "phidot_Z1_yaw"
  "p q r "/1 -> Reshape1/1
  Euler_angs/1 -> Demux1/1
  Demux3/1 -> euler_rates/3(p)
  Reshape2/1 -> Euler_rates/1
  Reshape1/1 -> Demux3/1  "wb"
  Demux3/3 -> euler_rates/5(r)
  Demux1/3 -> Terminator/1  "psi"
  euler_rates/1(euler_rates) -> Demux2/1  "euler_rates"
  Demux1/2 -> euler_rates/2(theta_t)  "theta"
  Mux1/1 -> Reshape2/1
  Demux2/3 -> Mux1/3  "psidot_X3_roll"

== system One_Sensor_Simulation/Quad with sensors/Integrate_quaternion/NORMLIZE_occasionally ==
  note: One strategy for NORMALIZING the quaternion
  note: eg: every 10 seconds normalize
  In1 : Inport
  Adjust_to_UNITY : Subsystem
  Out1 : Outport
  wires:
  In1/1 -> Adjust_to_UNITY/1(qin)
  Adjust_to_UNITY/1(q_unit) -> Out1/1

== system One_Sensor_Simulation/Quad_EOM/Integrate_quaternion/Calc Euler_rates ==
  "p q r " : Inport
  Euler_angs : Inport  Port=2
  Demux1 : Demux  Outputs=3
  Demux2 : Demux  Outputs=3
  Demux3 : Demux  Outputs=3
  Mux1 : Mux  Inputs=3
  Reshape1 : Reshape  OutputDimensionality=Column vector (2-D)
  Reshape2 : Reshape  OutputDimensionality=Column vector (2-D)
  Terminator : Terminator
  euler_rates : MATLAB Function  TreatAsAtomicUnit=on
  Euler_rates : Outport
  wires:
  Demux2/2 -> Mux1/2  "thetadot_Y2_pitch"
  Demux1/1 -> euler_rates/1(phi_t)  "phi"
  Demux3/2 -> euler_rates/4(q)
  Demux2/1 -> Mux1/1  "phidot_Z1_yaw"
  "p q r "/1 -> Reshape1/1
  Euler_angs/1 -> Demux1/1
  Demux3/1 -> euler_rates/3(p)
  Reshape2/1 -> Euler_rates/1
  Reshape1/1 -> Demux3/1  "wb"
  Demux3/3 -> euler_rates/5(r)
  Demux1/3 -> Terminator/1  "psi"
  euler_rates/1(euler_rates) -> Demux2/1  "euler_rates"
  Demux1/2 -> euler_rates/2(theta_t)  "theta"
  Mux1/1 -> Reshape2/1
  Demux2/3 -> Mux1/3  "psidot_X3_roll"

== system One_Sensor_Simulation/Quad_EOM/Integrate_quaternion/NORMLIZE_occasionally ==
  note: One strategy for NORMALIZING the quaternion
  note: eg: every 10 seconds normalize
  In1 : Inport
  Adjust_to_UNITY : Subsystem
  Out1 : Outport
  wires:
  In1/1 -> Adjust_to_UNITY/1(qin)
  Adjust_to_UNITY/1(q_unit) -> Out1/1

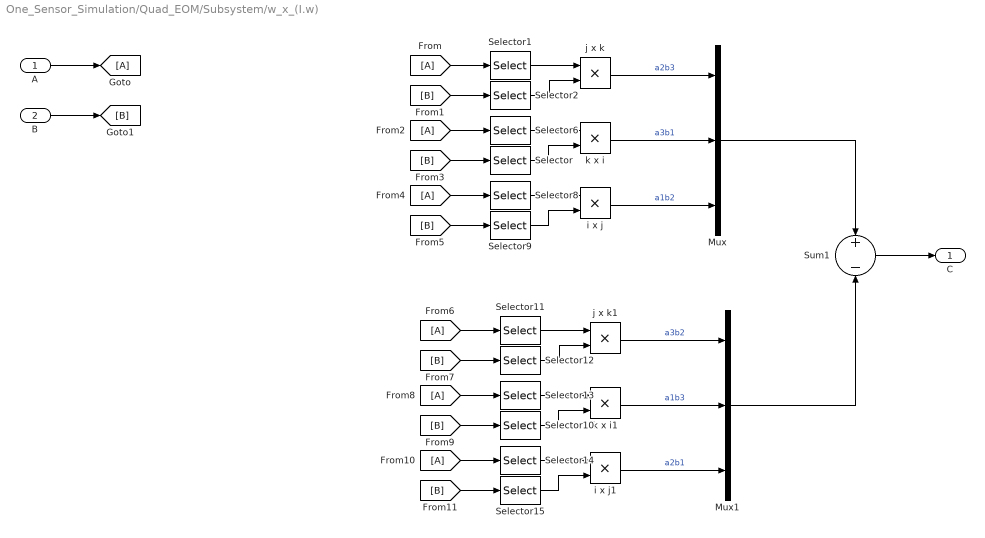
== system One_Sensor_Simulation/Quad_EOM/Subsystem/w_x_(I.w) ==
  A : Inport
  B : Inport  Port=2
  Mux : Mux  Inputs=3
  Mux1 : Mux  Inputs=3
  Selector{,8,13,15} (4 alike) : Selector  InputPortWidth=3  IndexOptions=Index vector (dialog)  Indices=1  OutputSizes=1
  Selector{1,9,12,14} (4 alike) : Selector  InputPortWidth=3  IndexOptions=Index vector (dialog)  Indices=2  OutputSizes=1
  Selector{2,6,10..11} (4 alike) : Selector  InputPortWidth=3  IndexOptions=Index vector (dialog)  Indices=3  OutputSizes=1
  Sum1 : Sum  Inputs=+|-  InputSameDT=on  SaturateOnIntegerOverflow=on  OutDataTypeStr=Inherit: Same as first input
  i x j : Product  InputSameDT=on  SaturateOnIntegerOverflow=on  OutDataTypeStr=Inherit: Same as first input
  i x j1 : Product  InputSameDT=on  SaturateOnIntegerOverflow=on  OutDataTypeStr=Inherit: Same as first input
  j x k : Product  InputSameDT=on  SaturateOnIntegerOverflow=on  OutDataTypeStr=Inherit: Same as first input
  j x k1 : Product  InputSameDT=on  SaturateOnIntegerOverflow=on  OutDataTypeStr=Inherit: Same as first input
  k x i : Product  InputSameDT=on  SaturateOnIntegerOverflow=on  OutDataTypeStr=Inherit: Same as first input
  k x i1 : Product  InputSameDT=on  SaturateOnIntegerOverflow=on  OutDataTypeStr=Inherit: Same as first input
  C : Outport
  wires:
  i x j/1 -> Mux/3  "a1b2"
  k x i/1 -> Mux/2  "a3b1"
  j x k/1 -> Mux/1  "a2b3"
  Mux/1 -> Sum1/1
  Sum1/1 -> C/1
  Selector1/1 -> j x k/1
  Selector2/1 -> j x k/2
  B/1 -> [B]
  A/1 -> [A]
  [B] -> Selector2/1
  [A] -> Selector1/1
  [A] -> Selector6/1
  [B] -> Selector/1
  Selector6/1 -> k x i/1
  Selector/1 -> k x i/2
  [A] -> Selector8/1
  [B] -> Selector9/1
  Selector8/1 -> i x j/1
  Selector9/1 -> i x j/2
  i x j1/1 -> Mux1/3  "a2b1"
  k x i1/1 -> Mux1/2  "a1b3"
  j x k1/1 -> Mux1/1  "a3b2"
  Mux1/1 -> Sum1/2
  Selector11/1 -> j x k1/1
  Selector12/1 -> j x k1/2
  [B] -> Selector12/1
  [A] -> Selector11/1
  [A] -> Selector13/1
  [B] -> Selector10/1
  Selector13/1 -> k x i1/1
  Selector10/1 -> k x i1/2
  [A] -> Selector14/1
  [B] -> Selector15/1
  Selector14/1 -> i x j1/1
  Selector15/1 -> i x j1/2
